simulink model "odev2 (1)"  (R2014a)
settings: Solver=ode45  StartTime=0.0  StopTime=10.0  RelTol=1e-3
undefined symbols (not defined in the file): gray, Rec, SDTV
libraries: visionconversions x4, visionsinks x2, visionsources x1, visionutilities x1
settings Model: Creator=bizimakin  LastModifiedBy=LENOVO
settings DebuggingCC: UnderspecifiedInitializationDetection=Classic  StateNameClashWarn=warning

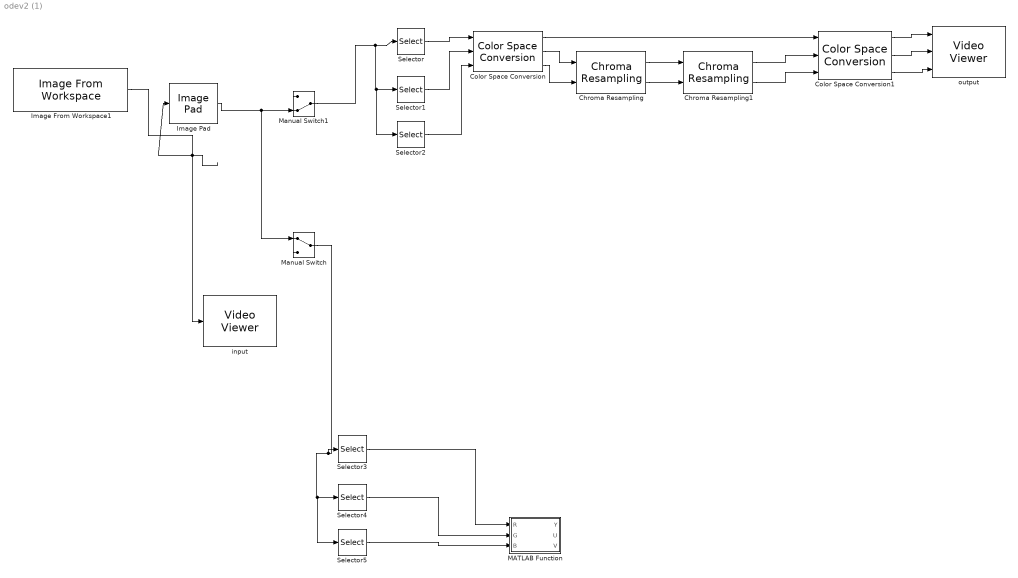
== system odev2 (1) ==
  Chroma Resampling : visionconversions/Chroma Resampling  resampling=4:4:4 to 4:2:2  interpolation=linear  antialiasing=Default  hcoeff=[0.2 0.6 0.2]  vcoeff=[0.5 0.5]  isInputTransposed=off
  Chroma Resampling1 : visionconversions/Chroma Resampling  resampling=4:2:2 to 4:4:4  interpolation=linear  antialiasing=Default  hcoeff=[0.2 0.6 0.2]  vcoeff=[0.5 0.5]  isInputTransposed=off
  Color Space Conversion : visionconversions/Color Space  Conversion  conversion=Obsolete  conversionActive=R'G'B' to Y'CbCr  wp_str=D65  rec=Rec. 601 (SDTV)  sys=1125/60/2:1  imagePorts=Separate color signals
  Color Space Conversion1 : visionconversions/Color Space  Conversion  conversion=Obsolete  conversionActive=Y'CbCr to R'G'B'  wp_str=D65  rec=Rec. 601 (SDTV)  sys=1125/60/2:1  imagePorts=Separate color signals
  Image From Workspace1 : visionsources/Image From Workspace  Tag=vipblks_nd  ImageValue=I  Ts=inf  imagePorts=One multidimensional signal  ImageDataType=Inherit from 'Value'  Signed=on  WordLength=16  sdImageDataType=sfix(16)  FractionLengthMode=User-defined  FractionLength=15  OutPortLabels=R|G|B
  Image Pad : visionutilities/Image Pad  method=Symmetric  valSrc=Input port  value=0  spec=Pad size  rowDirection=Right  outRowsMode=User-specified  rowSize=1  outColSize=10  colDirection=No padding  outColsMode=User-specified  colSize=[2 3]  outRowSize=12  trunc_flag=None
  MATLAB Function : MATLAB Function  TreatAsAtomicUnit=on
  Manual Switch : ManualSwitch
  Manual Switch1 : ManualSwitch  CurrentSetting=0
  Selector : Selector  NumberOfDimensions=3  InputPortWidth=3  IndexOptions=Select all,Select all,Index vector (dialog)  Indices=[1 3],1,1  OutputSizes=1,1,1
  Selector1 : Selector  NumberOfDimensions=3  InputPortWidth=3  IndexOptions=Select all,Select all,Index vector (dialog)  Indices=[1 3],1,2  OutputSizes=1,1,1
  Selector2 : Selector  NumberOfDimensions=3  InputPortWidth=3  IndexOptions=Select all,Select all,Index vector (dialog)  Indices=[1 3],1,3  OutputSizes=1,1,1
  Selector3 : Selector  NumberOfDimensions=3  InputPortWidth=3  IndexOptions=Select all,Select all,Index vector (dialog)  Indices=[1 3],1,1  OutputSizes=1,1,1
  Selector4 : Selector  NumberOfDimensions=3  InputPortWidth=3  IndexOptions=Select all,Select all,Index vector (dialog)  Indices=[1 3],1,2  OutputSizes=1,1,1
  Selector5 : Selector  NumberOfDimensions=3  InputPortWidth=3  IndexOptions=Select all,Select all,Index vector (dialog)  Indices=[1 3],1,3  OutputSizes=1,1,1
  input : visionsinks/Video Viewer  inputType=Obsolete7b  imagePorts=One multidimensional signal  useColorMap=off  colormapValue=gray(256)  specRange=off  minInputVal=0  maxInputVal=255  FigPos=[488 560 410 300]  AxisZoom=on  trueSizedOnce=off  OpenAtMdlStart=on  DefaultConfigurationName=vipscopes.VideoViewerScopeCfg
  output : visionsinks/Video Viewer  inputType=Obsolete7b  imagePorts=Separate color signals  useColorMap=off  colormapValue=gray(256)  specRange=off  minInputVal=0  maxInputVal=255  FigPos=[1023 557 410 300]  AxisZoom=on  trueSizedOnce=off  OpenAtMdlStart=on  DefaultConfigurationName=vipscopes.VideoViewerScopeCfg
  wires:
  Color Space Conversion/2 -> Chroma Resampling/1
  Color Space Conversion/1 -> Color Space Conversion1/1
  Color Space Conversion/3 -> Chroma Resampling/2
  Chroma Resampling/1 -> Chroma Resampling1/1
  Chroma Resampling/2 -> Chroma Resampling1/2
  Chroma Resampling1/1 -> Color Space Conversion1/2
  Chroma Resampling1/2 -> Color Space Conversion1/3
  Color Space Conversion1/1 -> output/1
  Color Space Conversion1/2 -> output/2
  Color Space Conversion1/3 -> output/3
  Image From Workspace1/1 -> Image Pad/1, input/1
  Manual Switch1/1 -> Selector2/1, Selector1/1, Selector/1
  Selector/1 -> Color Space Conversion/1
  Selector1/1 -> Color Space Conversion/2
  Selector2/1 -> Color Space Conversion/3
  Manual Switch/1 -> Selector5/1, Selector4/1, Selector3/1
  Selector3/1 -> MATLAB Function/1(R)
  Selector4/1 -> MATLAB Function/2(G)
  Selector5/1 -> MATLAB Function/3(B)
  Image Pad/1 -> Manual Switch/1, Manual Switch1/2

== matlab function odev2 (1)/MATLAB Function ==
  data: R input; G input; B input; Y output; U output; V output
function [Y,U,V] = fcn(R,G,B)


Y = 0.299 * R + 0.587 * G + 0.114 * B;
U = -0.14713 * R - 0.28886 * G + 0.436 * B;
V = 0.615 * R - 0.51499 * G - 0.10001 * B;
